simulink model "model"  (R2018a)
settings: Solver=FixedStepDiscrete  StartTime=0.0  StopTime=100  FixedStep=0.01  RelTol=1e-3
undefined symbols (not defined in the file): DiscIntNeverNeededParam
libraries: simulink_extras x1, discretizing x1, simulink x1
settings Model: Creator=Matteo  LastModifiedBy=Matteo

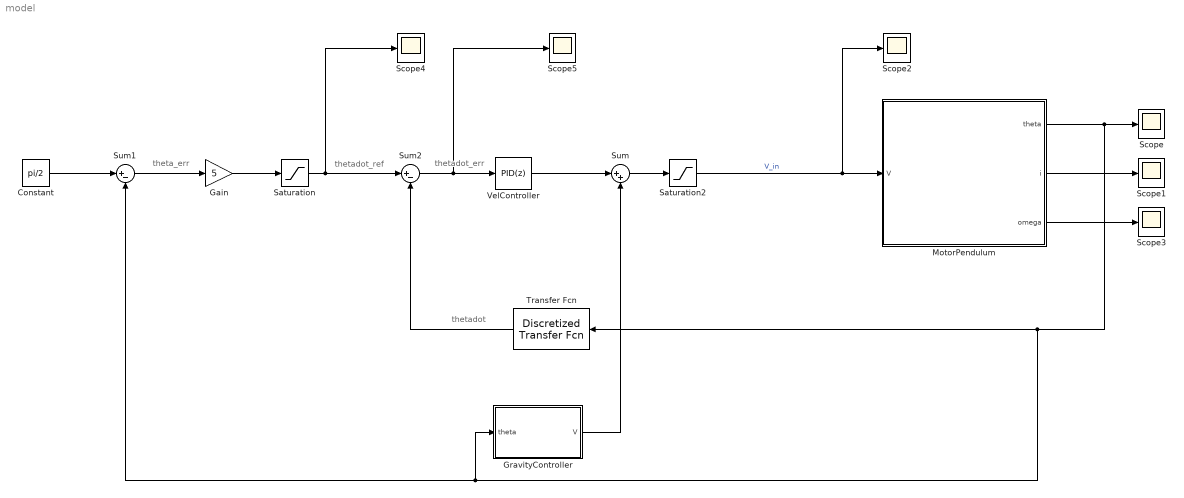
== system model ==
  note: thetadot_err
  note: theta_err
  note: thetadot_ref
  note: thetadot
  Constant : Constant  Value=pi/2
  Gain : Gain  Gain=5
  GravityController : Subsystem  mask{pwm90=200*24/4095, M=0.46700000, d=0.21666702, g=9.81, kt=0.08444, Kp=1.5, Kd=0, Ki=10}
      mask prompts: pwm90 "pwm at 90deg"; M "Mass"; d "distance CoM"; g "gravity accel"; kt "torque const"; Kp "proportional gain"; Kd "derivative gain"; Ki "integral gain"
  MotorPendulum : Subsystem  mask{R=0.174, L=0.076e-3, kv=0.08444, kt=0.08444, Im=0.0001380, Ip=0.00351785, M=0.163, d=0.109, g=9.81, theta0=0, thetad0=0}
      mask prompts: R "resistance"; L "inductance"; kv "velocity const [rad/s/V]"; kt "torque const [Nm/A]"; Im "Inertia motor"; Ip "Inertia pend"; M "Mass"; d "distance CoM"; g "gravity accel"; theta0 "theta initial"; thetad0 "w initial"
  Saturation : Saturate  UpperLimit=0.1  LowerLimit=-0.1
  Saturation2 : Saturate  UpperLimit=+10  LowerLimit=-10
  Scope{,1..5} (6 alike) : Scope
  Sum : Sum  Inputs=|++
  Sum1 : Sum  Inputs=|+-
  Sum2 : Sum  Inputs=|+-
  Transfer Fcn : discretizing/Discretized Transfer Fcn  Numerator=[1 0]  Denominator=[1/25 1]  AbsTol=auto  SampleTime=0.01  method=zoh  Wc=1
  VelController : simulink/Continuous/PID Controller  Controller=PID  TimeDomain=Discrete-time  SampleTime=-1  IntegratorMethod=Trapezoidal  FilterMethod=Trapezoidal  Form=Parallel  UseFilter=on  ControllerParametersSource=internal  P=5  I=1  D=0  N=182  InitialConditionSource=internal  InitialConditionForIntegrator=0  InitialConditionForFilter=0  ExternalReset=none  LimitOutput=off  UpperSaturationLimit=inf  LowerSaturationLimit=-inf  LinearizeAsGain=off  AntiWindupMode=none  Kb=1  TrackingMode=off  Kt=1  PParamMin=[]  PParamMax=[]  IParamMin=[]  IParamMax=[]  DParamMin=[]  DParamMax=[]  NParamMin=[]  NParamMax=[]  KbParamMin=[]  KbParamMax=[]  KtParamMin=[]  KtParamMax=[]  POutMin=[]  POutMax=[]  IOutMin=[]  IOutMax=[]  DOutMin=[]  DOutMax=[]  NOutMin=[]  NOutMax=[]  KbOutMin=[]  KbOutMax=[]  KtOutMin=[]  KtOutMax=[]  IntegratorOutMin=[]  IntegratorOutMax=[]  FilterOutMin=[]  FilterOutMax=[]  SumOutMin=[]  SumOutMax=[]  SumI1OutMin=[]  SumI1OutMax=[]  SumI2OutMin=[]  SumI2OutMax=[]  SumI3OutMin=[]  SumI3OutMax=[]  SumDOutMin=[]  SumDOutMax=[]  SaturationOutMin=[]  SaturationOutMax=[]  IntegratorContinuousStateAttributes=''  IntegratorStateMustResolveToSignalObject=off  IntegratorRTWStateStorageClass=Auto  FilterContinuousStateAttributes=''  FilterStateMustResolveToSignalObject=off  FilterRTWStateStorageClass=Auto  DifferentiatorICPrevScaledInput=0  DifferentiatorOutMin=[]  DifferentiatorOutMax=[]  FilterDiffOutCoefMin=[]  FilterDiffOutCoefMax=[]  SumDenOutMin=[]  SumDenOutMax=[]  SumNumOutMin=[]  SumNumOutMax=[]  ReciprocalOutMin=[]  ReciprocalOutMax=[]  DivideOutMin=[]  DivideOutMax=[]  TunerSelectOption=Transfer Function Based (PID Tuner App)
  wires:
  Gain/1 -> Saturation/1
  Saturation/1 -> Scope4/1, Sum2/1
  Transfer Fcn/1 -> Sum2/2
  Constant/1 -> Sum1/1
  Sum2/1 -> Scope5/1, VelController/1
  Sum1/1 -> Gain/1
  Sum/1 -> Saturation2/1
  VelController/1 -> Sum/1
  Saturation2/1 -> Scope2/1, MotorPendulum/1(V)  "V_in"
  MotorPendulum/1(theta) -> Transfer Fcn/1, Sum1/2, GravityController/1(theta), Scope/1
  MotorPendulum/2(i) -> Scope1/1
  MotorPendulum/3("omega ") -> Scope3/1
  GravityController/1(V) -> Sum/2

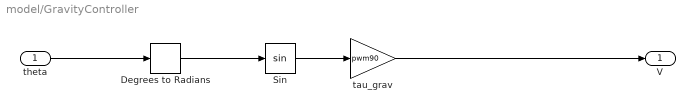
== system model/GravityController ==
  theta : Inport
  Degrees to Radians : simulink_extras/Transformations/Degrees to Radians
  Sin : Trigonometry
  tau_grav : Gain  Gain=pwm90
  V : Outport
  wires:
  Sin/1 -> tau_grav/1
  theta/1 -> Degrees to Radians/1
  Degrees to Radians/1 -> Sin/1
  tau_grav/1 -> V/1

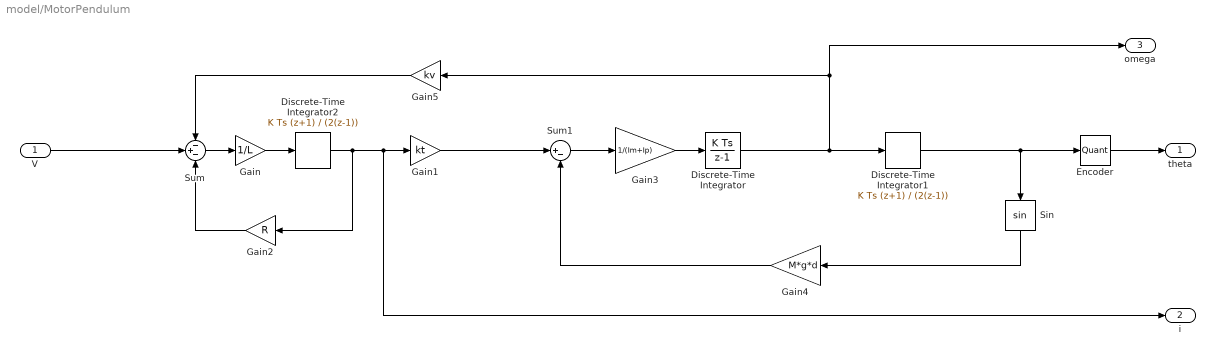
== system model/MotorPendulum ==
  V : Inport
  Discrete-Time Integrator : DiscreteIntegrator  InitialCondition=thetad0  SampleTime=-1  ICPrevOutput=DiscIntNeverNeededParam  ICPrevScaledInput=DiscIntNeverNeededParam
  Discrete-Time Integrator1 : DiscreteIntegrator  IntegratorMethod=Integration: Trapezoidal  InitialCondition=theta0  SampleTime=-1  ICPrevOutput=DiscIntNeverNeededParam  ICPrevScaledInput=DiscIntNeverNeededParam
  Discrete-Time Integrator2 : DiscreteIntegrator  IntegratorMethod=Integration: Trapezoidal  SampleTime=-1  ICPrevOutput=DiscIntNeverNeededParam  ICPrevScaledInput=DiscIntNeverNeededParam
  Encoder : Quantizer  QuantizationInterval=2*pi/2000
  Gain : Gain  Gain=1/L
  Gain1 : Gain  Gain=kt
  Gain2 : Gain  Gain=R
  Gain3 : Gain  Gain=1/(Im+Ip)
  Gain4 : Gain  Gain=M*g*d
  Gain5 : Gain  Gain=kv
  Sin : Trigonometry
  Sum : Sum  Inputs=-+-
  Sum1 : Sum  Inputs=|+-
  theta : Outport
  i : Outport  Port=2
  "omega " : Outport  Port=3
  wires:
  Gain3/1 -> Discrete-Time Integrator/1
  Gain4/1 -> Sum1/2
  V/1 -> Sum/2
  Gain/1 -> Discrete-Time Integrator2/1
  Discrete-Time Integrator1/1 -> Encoder/1, Sin/1
  Discrete-Time Integrator/1 -> Discrete-Time Integrator1/1, "omega "/1, Gain5/1
  Gain5/1 -> Sum/1
  Sum/1 -> Gain/1
  Sin/1 -> Gain4/1
  Gain2/1 -> Sum/3
  Gain1/1 -> Sum1/1
  Discrete-Time Integrator2/1 -> i/1, Gain1/1, Gain2/1
  Sum1/1 -> Gain3/1
  Encoder/1 -> theta/1
